simulink model "sample1_integrator"  (R2014b)
settings: Solver=ode45  StartTime=0.0  StopTime=10.0  RelTol=1e-3
settings Model: Creator=simoz  LastModifiedBy=Victor

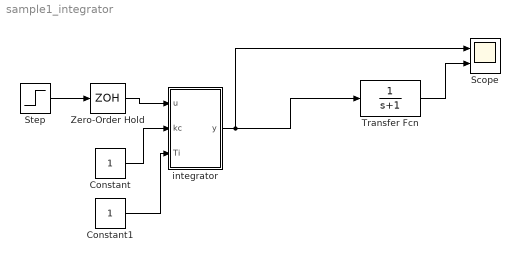
== system sample1_integrator ==
  Constant : Constant
  Constant1 : Constant
  Scope : Scope  NumInputPorts=2
      settings: YMin=0~0  YMax=1~1
  Step : Step  Time=0  After=5  SampleTime=0
  Transfer Fcn : TransferFcn  Denominator=[1 1]
  Zero-Order Hold : ZeroOrderHold  SampleTime=0.5
  "integrator " : MATLAB Function  TreatAsAtomicUnit=on
  wires:
  Transfer Fcn/1 -> Scope/2
  Zero-Order Hold/1 -> "integrator "/1(u)
  Step/1 -> Zero-Order Hold/1
  Constant/1 -> "integrator "/2(kc)
  Constant1/1 -> "integrator "/3(Ti)
  "integrator "/1(y) -> Scope/1, Transfer Fcn/1

== matlab function sample1_integrator/integrator  ==
  data: u input; y output; kc input; Ti input
function y = fcn(u, kc, Ti)

persistent I % статическая переменная

if isempty(I)
    I = 0;
end
I = I + u;

y = I;
